simulink model "FindPort"  (R2018b)
settings: Solver=VariableStepAuto  StartTime=0.0  StopTime=10.0  RelTol=1e-3
settings Model: Creator=dell  LastModifiedBy=dell
settings DebuggingCC: UnderSpecifiedDimensionMsg=warning

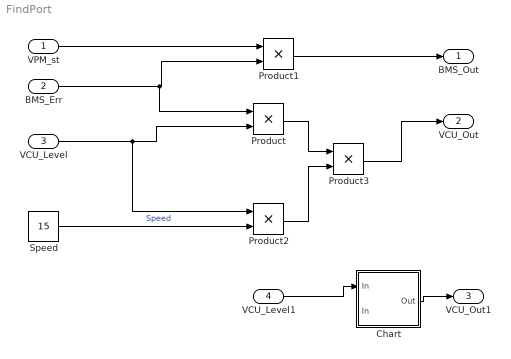
== system FindPort ==
  VPM_st : Inport
  BMS_Err : Inport  Port=2
  VCU_Level : Inport  Port=3
  VCU_Level1 : Inport  Port=4
  Chart : Stateflow chart  TreatAsAtomicUnit=on  SystemSampleTime=0.01
  Product{,1..3} (4 alike) : Product
  Speed : Constant  Value=15
  BMS_Out : Outport
  VCU_Out : Outport  Port=2
  VCU_Out1 : Outport  Port=3
  wires:
  VPM_st/1 -> Product1/1
  BMS_Err/1 -> Product/1, Product1/2
  VCU_Level/1 -> Product2/1, Product/2
  Product1/1 -> BMS_Out/1
  Speed/1 -> Product2/2  "Speed"
  Product/1 -> Product3/1
  Product2/1 -> Product3/2
  Product3/1 -> VCU_Out/1
  VCU_Level1/1 -> Chart/1(In)
  Chart/1(Out) -> VCU_Out1/1

== stateflow chart FindPort/Chart ==
  state START
    en:Out = ln;
  (default) -> START
  data: In input; Out output; ln input
